simulink model "rotary_pto_example"  (R2014a)
settings: Solver=ode45  StartTime=0.0  StopTime=10.0  RelTol=1e-3
undefined symbols (not defined in the file or in its folder): body, pcc_c, X, Y, Z
libraries: sm_lib x3, WECSim_Lib x2, nesl_utility x2
settings Model: Creator=kmruehl  LastModifiedBy=kmruehl
settings DebuggingCC: UnderspecifiedInitializationDetection=Classic  StateNameClashWarn=warning

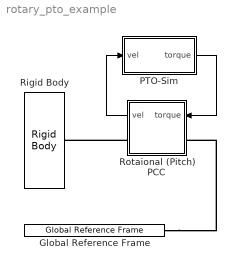
== system rotary_pto_example ==
  Global Reference Frame : WECSim_Lib/Frames/Global Reference Frame  waves=waves  simu=simu
  PTO-Sim : Subsystem
  Rigid Body : WECSim_Lib/Body Elements/Rigid Body  Coupling=No  body=body(1)
      settings: AttributesFormatString=%<body>
  Rotaional (Pitch) PCC : Subsystem  mask{pcc_k=0, pcc_c=0, pcc_connectionPoint=[0 0 0]}
      mask prompts: pcc_k "PTO stiffness"; pcc_c "PTO Damping Coe"; pcc_connectionPoint "Connection Location"
  wires:
  Rotaional (Pitch) PCC/1(vel) -> PTO-Sim/1(vel)
  PTO-Sim/1(torque) -> Rotaional (Pitch) PCC/1(torque)
  connections:
  Rotaional (Pitch) PCC/RConn1 -- Rigid Body/RConn1
  Global Reference Frame/RConn1 -- Rotaional (Pitch) PCC/LConn1

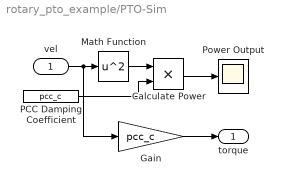
== system rotary_pto_example/PTO-Sim ==
  vel : Inport
  Calculate Power : Product  Inputs=**
  Gain : Gain  Gain=pcc_c
  Math Function : Math  Operator=square  SaturateOnIntegerOverflow=on
  PCC Damping Coefficient : Constant  Value=pcc_c
  Power Output : Scope
      settings: ShowLegends=on  YMin=0  YMax=15000  SaveName=ScopeData5
  torque : Outport
  wires:
  Calculate Power/1 -> Power Output/1
  Math Function/1 -> Calculate Power/1
  PCC Damping Coefficient/1 -> Calculate Power/2
  Gain/1 -> torque/1
  vel/1 -> Gain/1, Math Function/1

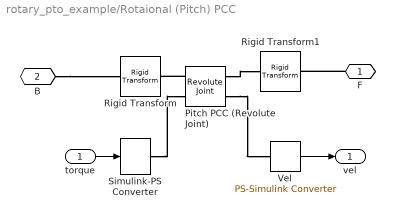
== system rotary_pto_example/Rotaional (Pitch) PCC ==
  torque : Inport
  Pitch PCC (Revolute Joint) : sm_lib/Joints/Revolute Joint  SenseConstraintForce=off  SenseConstraintForceX=off  SenseConstraintForceY=off  SenseConstraintForceZ=off  SenseConstraintTorque=off  SenseConstraintTorqueX=off  SenseConstraintTorqueY=off  SenseConstraintTorqueZ=off  SenseTotalForce=off  SenseTotalForceX=off  SenseTotalForceY=off  SenseTotalForceZ=off  SenseTotalTorque=off  SenseTotalTorqueX=off  SenseTotalTorqueY=off  SenseTotalTorqueZ=off  CompositeWrenchDir=FollowerOnBase  CompositeWrenchFrame=BaseFrame  EquilibriumPosition=0  EquilibriumPositionUnits=deg  SpringStiffness=0  SpringStiffnessUnits=N*m/deg  DampingCoefficient=pcc_c  DampingCoefficientUnits=N*m/(rad/s)  TorqueActuationMode=InputTorque  MotionActuationMode=ComputedMotion  SensePosition=off  SenseVelocity=on  SenseAcceleration=off  SenseTorqueForce=off  PositionTargetValue=0  PositionTargetValueUnits=deg  PositionTargetSpecify=off  PositionTargetPriority=High  VelocityTargetValue=0  VelocityTargetValueUnits=deg/s  VelocityTargetSpecify=off  VelocityTargetPriority=High  BlockFunction=simmechanics.library.joints.revolute_joint
  Rigid Transform : sm_lib/Frames and Transforms/Rigid Transform  TranslationMethod=Cartesian  TranslationLengthUnit=m  TranslationStandardAxis=+Z  TranslationStandardOffset=0  TranslationCartesianOffset=pcc_connectionPoint  TranslationROffset=0  TranslationROffsetUnits=m  TranslationZOffset=0  TranslationZOffsetUnits=m  TranslationThetaOffset=0  TranslationThetaOffsetUnits=deg  RotationMethod=StandardAxis  RotationAngleUnits=deg  RotationStandardAxis=+X  RotationAngle=90  RotationArbitraryAxis=[0 0 1]  FollAlignAxisA=+X  BaseAlignAxisA=+Y  FollAlignAxisB=+Y  BaseAlignAxisB=+Z  BlockFunction=simmechanics.library.frames_transforms.rigid_transform
  Rigid Transform1 : sm_lib/Frames and Transforms/Rigid Transform  TranslationMethod=Cartesian  TranslationLengthUnit=m  TranslationStandardAxis=+Z  TranslationStandardOffset=0  TranslationCartesianOffset=pcc_connectionPoint  TranslationROffset=0  TranslationROffsetUnits=m  TranslationZOffset=0  TranslationZOffsetUnits=m  TranslationThetaOffset=0  TranslationThetaOffsetUnits=deg  RotationMethod=StandardAxis  RotationAngleUnits=deg  RotationStandardAxis=+X  RotationAngle=90  RotationArbitraryAxis=[0 0 1]  FollAlignAxisA=+X  BaseAlignAxisA=+Y  FollAlignAxisB=+Y  BaseAlignAxisB=+Z  BlockFunction=simmechanics.library.frames_transforms.rigid_transform
  Simulink-PS Converter : nesl_utility/Simulink-PS Converter  PhysicalDomain=network_engine_domain  SubClassName=ps_input  LeftPortType=input  RightPortType=output  PseudoPeriodic=off  Frequencies=[]  NoiseDistribution=none  NoiseParameters=[]  Unit=1  AffineConversion=off  InputFiltering=off  SimscapeFilterOrder=1  InputFilterTimeConstant=0.001  UdotUserProvided=1
  Vel : nesl_utility/PS-Simulink Converter  PhysicalDomain=network_engine_domain  SubClassName=ps_output  LeftPortType=input  RightPortType=output  PseudoPeriodic=off  Frequencies=[]  Unit=1  AffineConversion=off
  F : PMIOPort  Port=1  Side=Right
  B : PMIOPort  Port=2  Side=Left
  vel : Outport
  wires:
  Vel/1 -> vel/1
  torque/1 -> Simulink-PS Converter/1
  connections:
  Pitch PCC (Revolute Joint)/LConn1 -- Rigid Transform/RConn1
  Pitch PCC (Revolute Joint)/RConn1 -- Rigid Transform1/RConn1
  Pitch PCC (Revolute Joint)/RConn2 -- Vel/LConn1
  B/RConn1 -- Rigid Transform/LConn1
  F/RConn1 -- Rigid Transform1/LConn1
  Simulink-PS Converter/RConn1 -- Pitch PCC (Revolute Joint)/LConn2
